simulink model "FOC"  (R2023a)
settings: Solver=ode1  StartTime=0.0  StopTime=0.2  FixedStep=ctrlConst.TsSwitch  MaxStep=1e-6  RelTol=1e-3  EnableMultiTasking=on
values from neighbouring files (symbols this model uses):
  f32_P_AngleCompCur = 5461.0    [bldc.sldd]
  f32_P_AngleCompVol = 1.5    [bldc.sldd]
  f32_P_IdInIF_A = -5.0    [bldc.sldd]
  f32_P_Modulation = 0.95    [bldc.sldd]
  u16_P_MotorPair = 4.0    [bldc.sldd]
undefined symbols (not defined in the file or in its folder): ECM, f32_P_Coef, FFW_enable, g_msgCore0to2_AcrKi, g_msgCore0to2_AcrKiStb, g_msgCore0to2_AcrKp, g_msgCore0to2_AcrKpStb, g_msgCore0to2_AcrSwtHiRpm, g_msgCore0to2_AcrSwtLoRpm, g_msgCore0to2_AfrKp, g_msgCore0to2_AfrTi, g_msgCore0to2_arc_dd_fi, g_msgCore0to2_CalibEn, g_msgCore0to2_clpwitch, g_msgCore0to2_DecoupleEn, g_msgCore0to2_dqLpf, g_msgCore0to2_dqLpfSpdCoef, g_msgCore0to2_FFW_Gain, g_msgCore0to2_linearKpEn, g_msgCore0to2_maxCur, g_msgCore0to2_maxFwcCurRatio, g_msgCore0to2_motorseq, g_msgCore0to2_MTPA_Gain, g_msgCore0to2_pwmFrqSet, g_msgCore0to2_spdswitch, IdROL_C, PWMFrqSwitch_C, SC_Ld_P, SC_Lq_P, SC_Psi_P, Tsw
libraries: MathLib x6, simulink x1
(part 2 of 2)

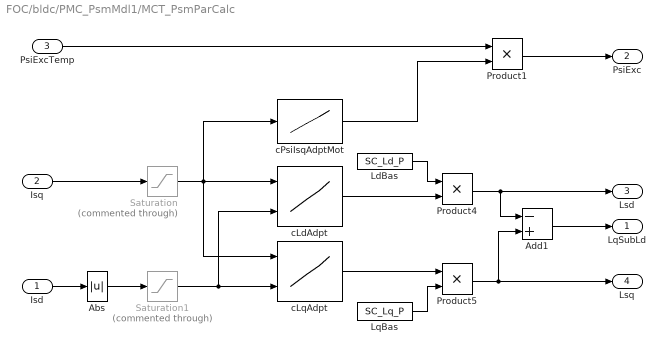
== system FOC/bldc/PMC_PsmMdl1/MCT_PsmParCalc ==
  Isd : Inport
  Isq : Inport  Port=2
  PsiExcTemp : Inport  Port=3
  Abs : Abs  SaturateOnIntegerOverflow=off
  Add1 : Sum  Inputs=-+
  LdBas : Constant  Value=SC_Ld_P  OutDataTypeStr=single  SampleTime=-1
  LqBas : Constant  Value=SC_Lq_P  OutDataTypeStr=single  SampleTime=-1
  Product1 : Product  OutDataTypeStr=single  RndMeth=Zero
  Product4 : Product  RndMeth=Zero  OutDataTypeStr=Inherit: Same as first input
  Product5 : Product  OutDataTypeStr=single  RndMeth=Zero
  Saturation : Saturate  Commented=through  UpperLimit=450  LowerLimit=-450
  Saturation1 : Saturate  Commented=through  UpperLimit=450  LowerLimit=0
  cLdAdpt : Lookup_n-D  DataSpecification=Lookup table object  LookupTableObject=cLdAdptMon_T  BreakpointsForDimension1=|  BreakpointsForDimension2=|  BeginIndexSearchUsingPreviousIndexResult=on  Table=|  ExtrapMethod=Clip  UseLastTableValue=on  InternalRulePriority=Speed  OutDataTypeStr=Inherit: Inherit from 'Table data'  InputSameDT=off
      BreakpointsForDimension1=|
      | [-530.4101839
      | -495.049505
      | -459.688826
      | -424.3281471
      | -388.9674682
      | -353.6067893
      | -318.2461103
      | -282.8854314
      | -247.5247525
      | -212.1640736
      | -176.8033946
      | -141.4427157
      | -106.0820368
      | -70.72135785
      | -35.36067893
      | 0
      | 35.36067893
      | 70.72135785
      | 106.0820368
      | 141.4427157
      | 176.8033946
      | 212.1640736
      | 247.5247525
      | 282.8854314
      | 318.2461103
      | 353.6067893
      | 388.9674682
      | 424.3281471
      | 459.688826
      | 495.049505
      | 530.4101839
      | ]
      BreakpointsForDimension2=|
      | [0	35.36067893	70.72135785	106.0820368	141.4427157	176.8033946	212.1640736	247.5247525	282.8854314	318.2461103	353.6067893	388.9674682	424.3281471	459.688826	495.049505	530.4101839
      | ]
      Table=|
      | [1	1	0.797297297	0.72972973	0.692567568	0.667567568	0.653153153	0.640926641	0.631756757	0.624624625	0.618918919	0.614742015	0.611486486	0.608731809	0.606177606	0.606177606
      | 1	1	0.797297297	0.72972973	0.692567568	0.667567568	0.653153153	0.640926641	0.631756757	0.624624625	0.618918919	0.614742015	0.611486486	0.608731809	0.606177606	0.606177606
      | 0.905405405	0.905405405	0.756756757	0.702702703	0.675675676	0.659459459	0.648648649	0.638996139	0.631756757	0.626126126	0.622972973	0.62002457	0.61768018	0.615800416	0.613899614	0.613899614
      | 0.810810811	0.810810811	0.716216216	0.68018018	0.665540541	0.651351351	0.644144144	0.638996139	0.633445946	0.630630631	0.628378378	0.626658477	0.625337838	0.624220374	0.622586873	0.622586873
      | 0.72972973	0.72972973	0.682432432	0.666666667	0.655405405	0.651351351	0.646396396	0.640926641	0.640202703	0.638138138	0.637027027	0.636240786	0.635585586	0.634927235	0.634169884	0.634169884
      | 0.635135135	0.635135135	0.648648649	0.648648649	0.648648649	0.648648649	0.646396396	0.646718147	0.64527027	0.645645646	0.646216216	0.646314496	0.646283784	0.646153846	0.645752896	0.645752896
      | 0.567567568	0.567567568	0.621621622	0.63963964	0.64527027	0.648648649	0.650900901	0.652509653	0.655405405	0.656606607	0.657837838	0.658562654	0.659009009	0.659043659	0.659266409	0.659266409
      | 0.513513514	0.513513514	0.601351351	0.630630631	0.64527027	0.654054054	0.65990991	0.664092664	0.665540541	0.67042042	0.672297297	0.673464373	0.674099099	0.674636175	0.673745174	0.673745174
      | 0.459459459	0.459459459	0.587837838	0.630630631	0.652027027	0.664864865	0.673423423	0.67953668	0.684121622	0.686786787	0.688918919	0.69017199	0.690653153	0.69022869	0.689189189	0.689189189
      | 0.432432432	0.432432432	0.587837838	0.63963964	0.668918919	0.683783784	0.695945946	0.702702703	0.706081081	0.709159159	0.710513514	0.713022113	0.710247748	0.708939709	0.707528958	0.707528958
      | 0.432432432	0.432432432	0.608108108	0.666666667	0.695945946	0.713513514	0.725225225	0.72972973	0.733108108	0.733483483	0.732986486	0.731572482	0.72972973	0.726611227	0.722972973	0.722972973
      | 0.486486486	0.486486486	0.662162162	0.716216216	0.743243243	0.754054054	0.761261261	0.760617761	0.760304054	0.758108108	0.755135135	0.751474201	0.747747748	0.742203742	0.737451737	0.737451737
      | 0.594594595	0.594594595	0.736486486	0.774774775	0.787162162	0.789189189	0.788288288	0.785714286	0.781756757	0.777027027	0.771891892	0.766093366	0.760135135	0.753638254	0.747104247	0.747104247
      | 0.72972973	0.72972973	0.804054054	0.81981982	0.820945946	0.818918919	0.813063063	0.806949807	0.8	0.792747748	0.78527027	0.777641278	0.77027027	0.761954262	0.754826255	0.754826255
      | 0.797297297	0.797297297	0.837837838	0.842342342	0.841216216	0.835135135	0.826576577	0.82046332	0.81097973	0.802012012	0.792837838	0.783783784	0.774774775	0.767151767	0.758687259	0.758687259
      | 0.790540541	0.790540541	0.834459459	0.84009009	0.837837838	0.832432432	0.82545045	0.818532819	0.809712838	0.800848348	0.791756757	0.782555283	0.774211712	0.766112266	0.757722008	0.757722008
      | 0.783783784	0.783783784	0.831081081	0.837837838	0.834459459	0.82972973	0.824324324	0.816602317	0.808445946	0.799684685	0.790675676	0.781326781	0.773648649	0.765072765	0.756756757	0.756756757
      | 0.689189189	0.689189189	0.783783784	0.806306306	0.810810811	0.810810811	0.806306306	0.801158301	0.794932432	0.788243243	0.781216216	0.773710074	0.765765766	0.758835759	0.751930502	0.751930502
      | 0.554054054	0.554054054	0.716216216	0.756756757	0.773648649	0.781081081	0.781531532	0.77992278	0.776013514	0.771921922	0.767162162	0.761793612	0.755630631	0.749480249	0.744208494	0.744208494
      | 0.418918919	0.418918919	0.628378378	0.693693694	0.726351351	0.743243243	0.75	0.752895753	0.752195946	0.750900901	0.748513514	0.745331695	0.742117117	0.737006237	0.732625483	0.732625483
      | 0.351351351	0.351351351	0.567567568	0.63963964	0.675675676	0.697297297	0.709459459	0.718146718	0.722972973	0.724024024	0.736459459	0.723587224	0.721846847	0.719334719	0.716216216	0.716216216
      | 0.351351351	0.351351351	0.547297297	0.612612613	0.64527027	0.664864865	0.677927928	0.687258687	0.694256757	0.697747748	0.7	0.701105651	0.701238739	0.700623701	0.698841699	0.698841699
      | 0.378378378	0.378378378	0.547297297	0.599099099	0.628378378	0.662162162	0.657657658	0.666023166	0.670608108	0.675375375	0.678378378	0.68034398	0.681418919	0.681912682	0.681467181	0.681467181
      | 0.405405405	0.405405405	0.547297297	0.594594595	0.618243243	0.632432432	0.641891892	0.646718147	0.652027027	0.656306306	0.659189189	0.661277641	0.662725225	0.663201663	0.664092664	0.664092664
      | 0.459459459	0.459459459	0.560810811	0.599099099	0.614864865	0.624324324	0.630630631	0.635135135	0.638513514	0.641141141	0.643648649	0.64546683	0.646734234	0.647609148	0.647683398	0.647683398
      | 0.513513514	0.513513514	0.587837838	0.608108108	0.614864865	0.618918919	0.623873874	0.625482625	0.628378378	0.629129129	0.631216216	0.632309582	0.633220721	0.633783784	0.634169884	0.634169884
      | 0.594594595	0.594594595	0.614864865	0.621621622	0.621621622	0.621621622	0.619369369	0.61969112	0.619932432	0.62012012	0.621081081	0.621498771	0.621734234	0.621933472	0.621621622	0.621621622
      | 0.675675676	0.675675676	0.641891892	0.635135135	0.628378378	0.624324324	0.619369369	0.617760618	0.614864865	0.614114114	0.612837838	0.612285012	0.611936937	0.611538462	0.611003861	0.611003861
      | 0.756756757	0.756756757	0.682432432	0.653153153	0.638513514	0.62972973	0.621621622	0.615830116	0.611486486	0.608108108	0.606351351	0.604545455	0.603502252	0.602494802	0.601640927	0.601640927
      | 0.851351351	0.851351351	0.716216216	0.675675676	0.652027027	0.635135135	0.623873874	0.615830116	0.609797297	0.605105105	0.601216216	0.598525799	0.596418919	0.594698545	0.593243243	0.593243243
      | 0.851351351	0.851351351	0.716216216	0.675675676	0.652027027	0.635135135	0.623873874	0.615830116	0.609797297	0.605105105	0.601216216	0.598525799	0.596418919	0.594698545	0.593243243	0.593243243
      | ]
      settings: InputPortMap=u0,u1
  cLqAdpt : Lookup_n-D  DataSpecification=Lookup table object  LookupTableObject=cLqAdptMon_T  BreakpointsForDimension1=|  BreakpointsForDimension2=|  BeginIndexSearchUsingPreviousIndexResult=on  Table=|  ExtrapMethod=Clip  UseLastTableValue=on  InternalRulePriority=Speed  OutDataTypeStr=Inherit: Inherit from 'Table data'  InputSameDT=off
      BreakpointsForDimension1=|
      | [-530.4101839
      | -495.049505
      | -459.688826
      | -424.3281471
      | -388.9674682
      | -353.6067893
      | -318.2461103
      | -282.8854314
      | -247.5247525
      | -212.1640736
      | -176.8033946
      | -141.4427157
      | -106.0820368
      | -70.72135785
      | -35.36067893
      | 0
      | 35.36067893
      | 70.72135785
      | 106.0820368
      | 141.4427157
      | 176.8033946
      | 212.1640736
      | 247.5247525
      | 282.8854314
      | 318.2461103
      | 353.6067893
      | 388.9674682
      | 424.3281471
      | 459.688826
      | 495.049505
      | 530.4101839
      | ]
      BreakpointsForDimension2=|
      | [0	35.36067893	70.72135785	106.0820368	141.4427157	176.8033946	212.1640736	247.5247525	282.8854314	318.2461103	353.6067893	388.9674682	424.3281471	459.688826	495.049505	530.4101839
      | ]
      Table=|
      | [0.394500897	0.39748954	0.39748954	0.400478183	0.403466826	0.403466826	0.403466826	0.406455469	0.406455469	0.406455469	0.403466826	0.403466826	0.403466826	0.400478183	0.400478183	0.400478183
      | 0.394500897	0.39748954	0.39748954	0.400478183	0.403466826	0.403466826	0.403466826	0.406455469	0.406455469	0.406455469	0.403466826	0.403466826	0.403466826	0.400478183	0.400478183	0.400478183
      | 0.418410042	0.421628581	0.424847119	0.424847119	0.428065658	0.428065658	0.428065658	0.428065658	0.431284197	0.428065658	0.428065658	0.428065658	0.424847119	0.424847119	0.421628581	0.421628581
      | 0.446304045	0.449790795	0.453277545	0.453277545	0.456764296	0.456764296	0.456764296	0.456764296	0.456764296	0.456764296	0.453277545	0.453277545	0.449790795	0.449790795	0.446304045	0.446304045
      | 0.479269684	0.483073412	0.483073412	0.48687714	0.48687714	0.48687714	0.48687714	0.48687714	0.48687714	0.48687714	0.483073412	0.483073412	0.479269684	0.475465957	0.471662229	0.471662229
      | 0.514644351	0.518828452	0.518828452	0.523012552	0.523012552	0.523012552	0.523012552	0.523012552	0.523012552	0.518828452	0.514644351	0.514644351	0.510460251	0.506276151	0.49790795	0.49790795
      | 0.557880056	0.562529056	0.562529056	0.562529056	0.562529056	0.562529056	0.562529056	0.562529056	0.557880056	0.557880056	0.553231055	0.548582055	0.543933054	0.534635053	0.529986053	0.529986053
      | 0.606694561	0.611924686	0.611924686	0.611924686	0.611924686	0.611924686	0.606694561	0.606694561	0.601464435	0.59623431	0.591004184	0.585774059	0.575313808	0.570083682	0.559623431	0.559623431
      | 0.669456067	0.669456067	0.669456067	0.669456067	0.669456067	0.663478781	0.663478781	0.657501494	0.651524208	0.639569635	0.633592349	0.621637776	0.61566049	0.603705918	0.593544531	0.593544531
      | 0.739191074	0.739191074	0.739191074	0.732217573	0.732217573	0.725244073	0.718270572	0.711297071	0.69735007	0.686889819	0.675034868	0.663179916	0.650627615	0.637377964	0.624825662	0.624825662
      | 0.816736402	0.815899582	0.812552301	0.806694561	0.79748954	0.785774059	0.772384937	0.758158996	0.743933054	0.728870293	0.713807531	0.69790795	0.682845188	0.667782427	0.652719665	0.652719665
      | 0.900627615	0.894351464	0.882845188	0.868200837	0.851464435	0.833682008	0.815899582	0.79707113	0.779288703	0.761506276	0.743723849	0.725941423	0.708158996	0.691422594	0.675732218	0.675732218
      | 0.965132497	0.949790795	0.928870293	0.907949791	0.885634589	0.864714086	0.845188285	0.824267782	0.80334728	0.782426778	0.762900976	0.741980474	0.723849372	0.705718271	0.688981869	0.688981869
      | 0.991631799	0.972803347	0.951882845	0.930962343	0.907949791	0.887029289	0.864016736	0.838912134	0.815899582	0.728033473	0.769874477	0.748953975	0.728033473	0.709205021	0.690376569	0.690376569
      | 1	0.979079498	0.958158996	0.937238494	0.920502092	0.89539749	0.866108787	0.841004184	0.811715481	0.786610879	0.757322176	0.736401674	0.715481172	0.690376569	0.673640167	0.673640167
      | 1	0.981171548	0.964435146	0.947698745	0.933054393	0.910041841	0.884937238	0.861924686	0.836820084	0.813807531	0.790794979	0.771966527	0.755230126	0.734309623	0.719665272	0.719665272
      | 1	0.983263598	0.970711297	0.958158996	0.945606695	0.924686192	0.90376569	0.882845188	0.861924686	0.841004184	0.824267782	0.807531381	0.794979079	0.778242678	0.765690377	0.765690377
      | 0.991631799	0.951882845	0.958158996	0.939330544	0.920502092	0.90167364	0.882845188	0.861924686	0.841004184	0.820083682	0.80125523	0.784518828	0.767782427	0.751046025	0.738493724	0.738493724
      | 0.965132497	0.951185495	0.933054393	0.913528591	0.894002789	0.875871688	0.857740586	0.839609484	0.820083682	0.80195258	0.783821478	0.767085077	0.750348675	0.735006974	0.719665272	0.719665272
      | 0.900627615	0.896443515	0.887029289	0.873430962	0.857740586	0.842050209	0.825313808	0.808577406	0.791841004	0.776150628	0.759414226	0.743723849	0.728033473	0.712343096	0.697698745	0.697698745
      | 0.816736402	0.817573222	0.815062762	0.810041841	0.80167364	0.791631799	0.779916318	0.767364017	0.753974895	0.739748954	0.725523013	0.711297071	0.69790795	0.683682008	0.670292887	0.670292887
      | 0.739191074	0.739191074	0.739191074	0.739191074	0.732217573	0.732217573	0.725244073	0.711297071	0.70432357	0.69525802	0.684797768	0.673640167	0.661785216	0.649930265	0.638075314	0.638075314
      | 0.669456067	0.669456067	0.669456067	0.669456067	0.669456067	0.669456067	0.663478781	0.657501494	0.657501494	0.645546922	0.639569635	0.633592349	0.621637776	0.61566049	0.603705918	0.603705918
      | 0.606694561	0.611924686	0.611924686	0.611924686	0.611924686	0.611924686	0.611924686	0.611924686	0.606694561	0.601464435	0.59623431	0.591004184	0.585774059	0.575313808	0.570083682	0.570083682
      | 0.557880056	0.562529056	0.562529056	0.567178057	0.567178057	0.567178057	0.567178057	0.562529056	0.562529056	0.557880056	0.557880056	0.553231055	0.548582055	0.543933054	0.539284054	0.539284054
      | 0.514644351	0.518828452	0.518828452	0.523012552	0.523012552	0.527196653	0.527196653	0.527196653	0.523012552	0.523012552	0.518828452	0.518828452	0.514644351	0.510460251	0.506276151	0.506276151
      | 0.479269684	0.479269684	0.483073412	0.48687714	0.48687714	0.490680867	0.490680867	0.490680867	0.490680867	0.490680867	0.48687714	0.48687714	0.483073412	0.479269684	0.475465957	0.475465957
      | 0.446304045	0.449790795	0.453277545	0.453277545	0.456764296	0.456764296	0.456764296	0.460251046	0.460251046	0.460251046	0.456764296	0.456764296	0.453277545	0.453277545	0.449790795	0.449790795
      | 0.418410042	0.421628581	0.424847119	0.424847119	0.428065658	0.428065658	0.431284197	0.431284197	0.431284197	0.431284197	0.431284197	0.431284197	0.428065658	0.428065658	0.424847119	0.424847119
      | 0.394500897	0.39748954	0.39748954	0.400478183	0.403466826	0.403466826	0.406455469	0.406455469	0.406455469	0.406455469	0.406455469	0.406455469	0.406455469	0.403466826	0.403466826	0.403466826
      | 0.394500897	0.39748954	0.39748954	0.400478183	0.403466826	0.403466826	0.406455469	0.406455469	0.406455469	0.406455469	0.406455469	0.406455469	0.406455469	0.403466826	0.403466826	0.403466826
      | ]
      settings: InputPortMap=u0,u1
  cPsiIsqAdptMot : Lookup_n-D  NumberOfTableDimensions=1  DataSpecification=Lookup table object  LookupTableObject=cPsiIsqAdptMot_TT  BreakpointsForDimension1=|  BeginIndexSearchUsingPreviousIndexResult=on  Table=|  ExtrapMethod=Clip  UseLastTableValue=on  InternalRulePriority=Speed  OutDataTypeStr=Inherit: Inherit from 'Table data'
      BreakpointsForDimension1=|
      | [-530.4101839
      | -495.049505
      | -459.688826
      | -424.3281471
      | -388.9674682
      | -353.6067893
      | -318.2461103
      | -282.8854314
      | -247.5247525
      | -212.1640736
      | -176.8033946
      | -141.4427157
      | -106.0820368
      | -70.72135785
      | -35.36067893
      | 0
      | 35.36067893
      | 70.72135785
      | 106.0820368
      | 141.4427157
      | 176.8033946
      | 212.1640736
      | 247.5247525
      | 282.8854314
      | 318.2461103
      | 353.6067893
      | 388.9674682
      | 424.3281471
      | 459.688826
      | 495.049505
      | 530.4101839
      | ]
      Table=|
      | [0.983333333
      | 0.983333333
      | 0.985185185
      | 0.987037037
      | 0.990740741
      | 0.992592593
      | 0.994444444
      | 0.996296296
      | 0.996296296
      | 0.998148148
      | 0.998148148
      | 0.998148148
      | 0.994444444
      | 0.992592593
      | 0.990740741
      | 0.990740741
      | 0.990740741
      | 0.992592593
      | 0.996296296
      | 1
      | 1
      | 1
      | 1
      | 0.998148148
      | 0.996296296
      | 0.994444444
      | 0.992592593
      | 0.990740741
      | 0.988888889
      | 0.987037037
      | 0.987037037]
  LqSubLd : Outport  VectorParamsAs1DForOutWhenUnconnected=off
  PsiExc : Outport  Port=2  VectorParamsAs1DForOutWhenUnconnected=off
  Lsd : Outport  Port=3  VectorParamsAs1DForOutWhenUnconnected=off
  Lsq : Outport  Port=4  VectorParamsAs1DForOutWhenUnconnected=off
  wires:
  PsiExcTemp/1 -> Product1/1
  Add1/1 -> LqSubLd/1
  Product5/1 -> Add1/2, Lsq/1
  Product4/1 -> Add1/1, Lsd/1
  Product1/1 -> PsiExc/1
  LqBas/1 -> Product5/2
  cLqAdpt/1 -> Product5/1
  cLdAdpt/1 -> Product4/2
  LdBas/1 -> Product4/1
  Abs/1 -> Saturation1/1
  Isq/1 -> Saturation/1
  Isd/1 -> Abs/1
  cPsiIsqAdptMot/1 -> Product1/2
  Saturation/1 -> cLqAdpt/1, cLdAdpt/1, cPsiIsqAdptMot/1
  Saturation1/1 -> cLqAdpt/2, cLdAdpt/2

== system FOC/bldc/PMC_PsmMdl1/PMC_TrqCal ==
  PMC_LqSubLd : Inport
  PMC_PsiExc : Inport  Port=2
  MCT_isdFlt : Inport  Port=3
  MCT_isqFlt : Inport  Port=4
  Constant : Constant  Value=500  OutDataTypeStr=single
  Gain1 : Gain  Gain=3*u16_P_MotorPair
  Gain2 : Gain  Gain=-1  ParamDataTypeStr=single
  Product : Product
  Product1 : Product
  Product2 : Product
  Saturation Dynamic1 : simulink/Discontinuities/Saturation Dynamic  OutMin=[]  OutMax=[]  OutDataTypeStr=Inherit: Same as second input  OutDataType=fixdt(1, 16)  OutScaling=2^-10  DoSatur=off
  Sum : Sum  Inputs=|+-
  MCT_TrqAct : Outport  VectorParamsAs1DForOutWhenUnconnected=off
  wires:
  Saturation Dynamic1/1 -> MCT_TrqAct/1
  Gain1/1 -> Saturation Dynamic1/2
  Constant/1 -> Saturation Dynamic1/1, Gain2/1
  Gain2/1 -> Saturation Dynamic1/3
  Sum/1 -> Gain1/1
  MCT_isqFlt/1 -> Product/2, Product2/1
  PMC_PsiExc/1 -> Product/1
  Product/1 -> Sum/1
  PMC_LqSubLd/1 -> Product1/2
  MCT_isdFlt/1 -> Product1/1
  Product1/1 -> Product2/2
  Product2/1 -> Sum/2

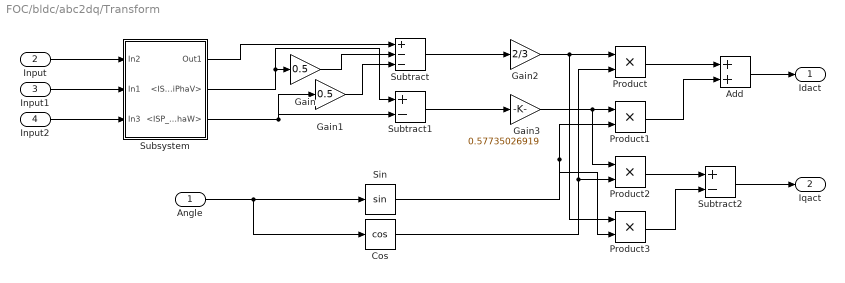
== system FOC/bldc/abc2dq/Transform ==
  Angle : Inport
  Input : Inport  Port=2
  Input1 : Inport  Port=3
  Input2 : Inport  Port=4
  Add : Sum  OutDataTypeStr=single
  Cos : Trigonometry  Operator=cos  OutputSignalType=real
  Gain : Gain  Gain=0.5
  Gain1 : Gain  Gain=0.5
  Gain2 : Gain  Gain=2/3
  Gain3 : Gain  Gain=0.57735026919
  Product{,1..3} (4 alike) : Product
  Sin : Trigonometry
  Subsystem : Subsystem
  Subtract : Sum  Inputs=+--
  Subtract1 : Sum  Inputs=+-
  Subtract2 : Sum  Inputs=+-  OutDataTypeStr=single
  Idact : Outport
  Iqact : Outport  Port=2
  wires:
  Subsystem/1(Out1) -> Subtract/1
  Subsystem/2(<ISP_iPhaV>) -> Subtract1/1, Gain/1
  Subsystem/3(<ISP_iPhaW>) -> Gain1/1, Subtract1/2
  Gain/1 -> Subtract/2
  Gain1/1 -> Subtract/3
  Subtract/1 -> Gain2/1
  Subtract1/1 -> Gain3/1
  Gain2/1 -> Product3/1, Product/1
  Cos/1 -> Product2/2, Product/2
  Product/1 -> Add/1
  Gain3/1 -> Product2/1, Product1/1
  Product1/1 -> Add/2
  Add/1 -> Idact/1
  Product2/1 -> Subtract2/1
  Product3/1 -> Subtract2/2
  Subtract2/1 -> Iqact/1
  Angle/1 -> Sin/1, Cos/1
  Sin/1 -> Product3/2, Product1/2
  Input1/1 -> Subsystem/2(In1)
  Input/1 -> Subsystem/1(In2)
  Input2/1 -> Subsystem/3(In3)

== system FOC/bldc/PMC_IsDesCalc/FWC/PI ==
  error : Inport
  Ts : Inport  Port=2
  Constant : Constant  Value=0.25  OutDataTypeStr=single
  Constant1 : Constant  Value=g_msgCore0to2_AfrKp
  Constant2 : Constant  Value=1.0  OutDataTypeStr=single
  Constant4 : Constant  Value=g_msgCore0to2_maxCur  OutDataTypeStr=single
  Constant5 : Constant  Value=g_msgCore0to2_AfrTi
  Constant6 : Constant  Value=0  OutDataTypeStr=single
  Divide : Product  Inputs=**  OutDataTypeStr=single
  Divide1 : Product  Inputs=**/  OutDataTypeStr=single
  Divide2 : Product  Inputs=**  OutDataTypeStr=single
  Divide3 : Product  Inputs=**  OutDataTypeStr=single
  Switch : Switch  Criteria=u2 > Threshold  SaturateOnIntegerOverflow=off  InputSameDT=off
  Switch2 : Switch  Criteria=u2 ~= 0  SaturateOnIntegerOverflow=off  InputSameDT=off
  Kp : Outport  VectorParamsAs1DForOutWhenUnconnected=off
  Ki : Outport  Port=2  VectorParamsAs1DForOutWhenUnconnected=off
  wires:
  Constant/1 -> Switch/1
  error/1 -> Switch/2
  Constant1/1 -> Divide/1
  Constant4/1 -> Divide/2
  Divide/1 -> Divide2/1, Divide1/1
  Ts/1 -> Divide1/2
  Constant5/1 -> Switch2/2, Divide1/3
  Divide1/1 -> Switch2/1
  Constant6/1 -> Switch2/3
  Switch2/1 -> Divide3/1
  Constant2/1 -> Switch/3
  Switch/1 -> Divide3/2, Divide2/2
  Divide2/1 -> Kp/1
  Divide3/1 -> Ki/1

== system FOC/bldc/PMC_IsDesCalc/MaxI vs Freq/PT1_2 ==
  bin : Inport
  cof : Inport  Port=2
  Constant : Constant  OutDataTypeStr=single
  Product1 : Product  RndMeth=Zero  OutDataTypeStr=Inherit: Same as first input
  Product3 : Product  RndMeth=Zero  OutDataTypeStr=Inherit: Same as first input
  Subtract : Sum  Inputs=-+  OutDataTypeStr=Inherit: Same as first input
  Sum1 : Sum  Inputs=|++  OutDataTypeStr=Inherit: Same as first input
  Unit Delay1 : UnitDelay  SampleTime=-1  HasFrameUpgradeWarning=on
  bout : Outport  VectorParamsAs1DForOutWhenUnconnected=off
  wires:
  Subtract/1 -> Product3/2
  Sum1/1 -> Unit Delay1/1, bout/1
  cof/1 -> Product1/2, Subtract/1
  Constant/1 -> Subtract/2
  bin/1 -> Product1/1
  Product1/1 -> Sum1/1
  Unit Delay1/1 -> Product3/1
  Product3/1 -> Sum1/2

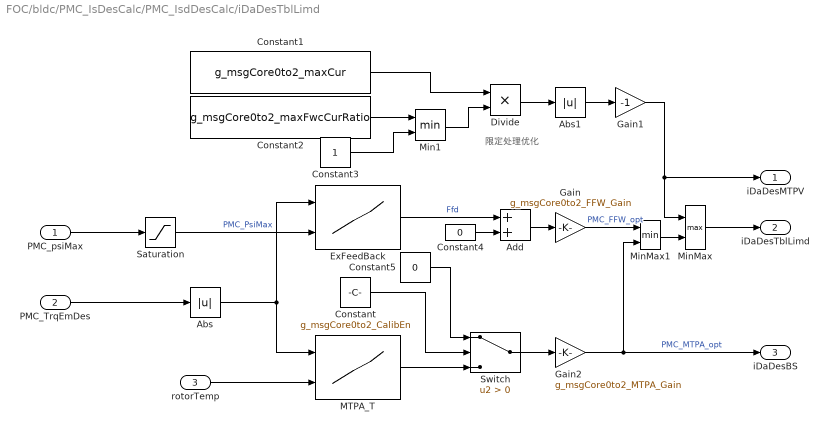
== system FOC/bldc/PMC_IsDesCalc/PMC_IsdDesCalc/iDaDesTblLimd ==
  note: 限定处理优化
  PMC_psiMax : Inport
  PMC_TrqEmDes : Inport  Port=2
  rotorTemp : Inport  Port=3
  Abs : Abs  SaturateOnIntegerOverflow=off
  Abs1 : Abs  OutDataTypeStr=single  SaturateOnIntegerOverflow=off
  Add : Sum
  Constant : Constant  Value=g_msgCore0to2_CalibEn
  Constant1 : Constant  Value=g_msgCore0to2_maxCur  OutDataTypeStr=single
  Constant2 : Constant  Value=g_msgCore0to2_maxFwcCurRatio  OutDataTypeStr=single
  Constant3 : Constant  OutDataTypeStr=single
  Constant4 : Constant  Value=0  OutDataTypeStr=single  SampleTime=-1
  Constant5 : Constant  Value=0  OutDataTypeStr=single
  Divide : Product  Inputs=**  OutDataTypeStr=single
  ExFeedBack : Lookup_n-D  DataSpecification=Lookup table object  LookupTableObject=ExFeedBack_T  BreakpointsForDimension1=|  BreakpointsForDimension2=|  BeginIndexSearchUsingPreviousIndexResult=on  Table=|  ExtrapMethod=Clip  UseLastTableValue=on  InternalRulePriority=Speed  OutDataTypeStr=Inherit: Inherit from 'Table data'  RndMeth=Simplest
      BreakpointsForDimension1=|
      | [0.015
      | 0.02
      | 0.025
      | 0.03
      | 0.035
      | 0.04
      | 0.06
      | 0.09]
      Table=|
      | [-180	-205	-250	-325	-340	-340	-340	-340	-340	-340	-340	-340	-340	-340	-340	-340	-340	-340	-340	-340	-340
      | -140	-160	-200	-255	-325	-340	-340	-340	-340	-340	-340	-340	-340	-340	-340	-340	-340	-340	-340	-340	-340
      | -100	-120	-160	-205	-275	-325	-340	-340	-340	-340	-340	-340	-340	-340	-340	-340	-340	-340	-340	-340	-340
      | -55	-80	-125	-170	-215	-280	-325	-340	-340	-340	-340	-340	-340	-340	-340	-340	-340	-340	-340	-340	-340
      | -20	-50	-90	-135	-180	-230	-295	-340	-340	-340	-340	-340	-340	-340	-340	-340	-340	-340	-340	-340	-340
      | -10	-20	-65	-105	-150	-190	-230	-280	-325	-340	-340	-340	-340	-340	-340	-340	-340	-340	-340	-340	-340
      | 0	-10	-30	-47	-60	-80	-115	-150	-180	-215	-245	-290	-325	-340	-340	-340	-340	-340	-340	-340	-340
      | 0	-10	-30	-47	-60	-78	-98	-113	-132	-152	-172	-194	-214	-228	-247	-271	-291	-315	-340	-340	-340
      | ]
      BreakpointsForDimension2=|
      | [0	20	40	60	80	100	120	140	160	180	200	220	240	260	280	300	320	340	360	380	400
      | ]
      settings: InputPortMap=u0,u1
  Gain : Gain  Gain=g_msgCore0to2_FFW_Gain
  Gain1 : Gain  Gain=-1  OutDataTypeStr=single
  Gain2 : Gain  Gain=g_msgCore0to2_MTPA_Gain
  MTPA_T : Lookup_n-D  DataSpecification=Lookup table object  LookupTableObject=MTPA_T  BreakpointsForDimension1=|  BreakpointsForDimension2=|  BeginIndexSearchUsingPreviousIndexResult=on  Table=|  ExtrapMethod=Clip  UseLastTableValue=on  InternalRulePriority=Speed  OutDataTypeStr=Inherit: Inherit from 'Table data'  RndMeth=Simplest
      BreakpointsForDimension1=|
      | [0
      | 20
      | 40
      | 60
      | 80
      | 100
      | 120
      | 140
      | 160
      | 180
      | 200
      | 220
      | 240
      | 260
      | 280
      | 300
      | 320
      | 340
      | 360
      | 380
      | 400]
      Table=|
      | [0.0 	0.0 	0.0 	0.0 	0.0 	0.0 	0.0 
      | -11.0 	-12.0 	-13.0 	-14.1 	-15.1 	-16.2 	-17.0 
      | -21.0 	-23.2 	-25.4 	-27.6 	-29.8 	-32.2 	-34.0 
      | -35.0 	-37.5 	-40.1 	-44.0 	-45.2 	-48.0 	-50.0 
      | -50.0 	-52.9 	-55.8 	-58.6 	-61.5 	-64.7 	-67.0 
      | -61.0 	-65.2 	-69.5 	-72.0 	-77.9 	-82.6 	-86.0 
      | -75.0 	-79.9 	-84.8 	-89.7 	-94.7 	-100.1 	-104.0 
      | -89.0 	-95.1 	-101.2 	-107.0 	-113.4 	-120.1 	-125.0 
      | -104.0 	-111.1 	-118.2 	-125.4 	-132.5 	-140.3 	-146.0 
      | -123.0 	-129.9 	-136.9 	-145.0 	-150.8 	-158.4 	-164.0 
      | -141.0 	-150.0 	-157.0 	-164.0 	-170.1 	-179.0 	-184.0 
      | -160.0 	-168.0 	-175.9 	-185.0 	-191.9 	-200.6 	-207.0 
      | -179.0 	-187.5 	-195.9 	-204.4 	-212.9 	-222.2 	-229.0 
      | -193.0 	-202.7 	-212.3 	-222.0 	-231.6 	-242.3 	-250.0 
      | -212.0 	-222.0 	-232.0 	-242.0 	-252.0 	-263.0 	-271.0 
      | -230.0 	-241.0 	-252.0 	-257.0 	-274.1 	-286.2 	-295.0 
      | -248.0 	-259.7 	-271.4 	-279.0 	-294.8 	-307.7 	-317.0 
      | -269.0 	-280.0 	-289.0 	-301.0 	-317.0 	-334.0 	-342.0 
      | -288.0 	-300.5 	-313.1 	-327.0 	-342.0 	-352.0 	-362.0 
      | -303.0 	-316.7 	-330.5 	-348.0 	-357.9 	-373.0 	-384.0 
      | -320.0 	-335.3 	-350.5 	-372.0 	-381.0 	-397.8 	-410.0 ]
      BreakpointsForDimension2=|
      | [-40	0	40	80	120	160	180
      | ]
      settings: InputPortMap=u0,u1
  Min1 : MinMax  Inputs=2
  MinMax : MinMax  Function=max  Inputs=2
  MinMax1 : MinMax  Inputs=2
  Saturation : Saturate  UpperLimit=0.18  LowerLimit=0.006
  Switch : Switch  Criteria=u2 > Threshold  SaturateOnIntegerOverflow=off  InputSameDT=off
  iDaDesMTPV : Outport  VectorParamsAs1DForOutWhenUnconnected=off
  iDaDesTblLimd : Outport  Port=2  VectorParamsAs1DForOutWhenUnconnected=off
  iDaDesBS : Outport  Port=3  VectorParamsAs1DForOutWhenUnconnected=off
  wires:
  Gain1/1 -> MinMax/1, iDaDesMTPV/1
  Constant4/1 -> Add/2
  ExFeedBack/1 -> Add/1  "Ffd"
  Switch/1 -> Gain2/1
  PMC_TrqEmDes/1 -> Abs/1
  MinMax/1 -> iDaDesTblLimd/1
  MinMax1/1 -> MinMax/2
  Saturation/1 -> ExFeedBack/2  "PMC_PsiMax"
  PMC_psiMax/1 -> Saturation/1
  Abs/1 -> ExFeedBack/1, MTPA_T/1
  rotorTemp/1 -> MTPA_T/2
  Divide/1 -> Abs1/1
  Constant1/1 -> Divide/1
  Abs1/1 -> Gain1/1
  Constant3/1 -> Min1/2
  Min1/1 -> Divide/2
  Constant2/1 -> Min1/1
  Constant/1 -> Switch/2
  MTPA_T/1 -> Switch/3
  Constant5/1 -> Switch/1
  Add/1 -> Gain/1
  Gain/1 -> MinMax1/1  "PMC_FFW_opt"
  Gain2/1 -> MinMax1/2, iDaDesBS/1  "PMC_MTPA_opt"

== system FOC/bldc/PMC_IsDesCalc/PMC_IsqDesCalc/IsqDesLim_Calc ==
  IsqTrqDes : Inport
  MCT_IsdDes : Inport  Port=2
  MCT_sgnTrqEmDes : Inport  Port=3
  Ismax : Inport  Port=4
  IsResDes : Constant  Value=0  OutDataTypeStr=single  SampleTime=-1
  Math Function : Math  Operator=square  SignedPower=on
  Math Function1 : Math  Operator=square  SignedPower=on
  Math Function2 : Math  Operator=square  SignedPower=on
  Product : Product  Inputs=**  RndMeth=Zero
  Relational Operator : RelationalOperator  Operator=<=  OutDataTypeStr=boolean  InputSameDT=off
  SQRT : Subsystem
  Sum1 : Sum  Inputs=|+-
  Sum2 : Sum  Inputs=|+-
  bIsResLimActv : Outport  VectorParamsAs1DForOutWhenUnconnected=off
  IsqDesLim : Outport  Port=2  VectorParamsAs1DForOutWhenUnconnected=off
  wires:
  Product/1 -> IsqDesLim/1
  Relational Operator/1 -> SQRT/Enable, bIsResLimActv/1
  MCT_sgnTrqEmDes/1 -> Product/2
  SQRT/1(Sqrt1) -> Product/1
  Sum1/1 -> SQRT/1(x), Sum2/1
  IsResDes/1 -> Relational Operator/2
  Sum2/1 -> Relational Operator/1
  Math Function2/1 -> Sum2/2
  Math Function1/1 -> Sum1/2
  Math Function/1 -> Sum1/1
  IsqTrqDes/1 -> Math Function2/1
  MCT_IsdDes/1 -> Math Function1/1
  Ismax/1 -> Math Function/1

== system FOC/bldc/PMC_IsDesCalc/PMC_IsqDesCalc/IsqTrqDes_Calc ==
  MCT_TrqEmDes : Inport
  MCT_IsdDes : Inport  Port=2
  MCT_LqSubLd : Inport  Port=3
  MCT_PsiExc : Inport  Port=4
  Constant10 : Constant  Value=g_msgCore0to2_CalibEn
  MCT_PsmPsiTrqCalc : Subsystem
  MCT_TrqEmLos : Constant  Value=0  OutDataTypeStr=single
  Product : Product  Inputs=*/  RndMeth=Zero
  Sum3 : Sum  Inputs=|+-
  Switch : Switch  Criteria=u2 > Threshold  SaturateOnIntegerOverflow=off  InputSameDT=off
  IsqTrqDes : Outport  VectorParamsAs1DForOutWhenUnconnected=off
  LqsubLdId : Outport  Port=2
  psi : Outport  Port=3
  wires:
  MCT_IsdDes/1 -> MCT_PsmPsiTrqCalc/1(MCT_IsdDes)
  MCT_PsiExc/1 -> MCT_PsmPsiTrqCalc/3(MCT_PsiExc)
  MCT_LqSubLd/1 -> MCT_PsmPsiTrqCalc/2(MCT_LqSubLd)
  MCT_TrqEmLos/1 -> Sum3/2
  MCT_TrqEmDes/1 -> Sum3/1
  MCT_PsmPsiTrqCalc/1(psiMul3p) -> Product/2
  Constant10/1 -> Switch/2
  Switch/1 -> IsqTrqDes/1
  Product/1 -> Switch/3
  Sum3/1 -> Switch/1, Product/1
  MCT_PsmPsiTrqCalc/2(LqsubLdId) -> LqsubLdId/1
  MCT_PsmPsiTrqCalc/3(psi) -> psi/1

== system FOC/bldc/abc2dq/Transform/Subsystem ==
  In2 : Inport
  In1 : Inport  Port=2
  In3 : Inport  Port=3
  Constant : Constant  Value=g_msgCore0to2_motorseq  OutDataTypeStr=uint16
  Switch : Switch  Criteria=u2 > Threshold  SaturateOnIntegerOverflow=off  InputSameDT=off
  Switch1 : Switch  Criteria=u2 > Threshold  SaturateOnIntegerOverflow=off  InputSameDT=off
  Out1 : Outport
  <ISP_iPhaV> : Outport  Port=2
  <ISP_iPhaW> : Outport  Port=3
  wires:
  In2/1 -> Out1/1
  In1/1 -> Switch/3, Switch1/1
  Switch1/1 -> <ISP_iPhaV>/1
  In3/1 -> Switch1/3, Switch/1
  Constant/1 -> Switch/2, Switch1/2
  Switch/1 -> <ISP_iPhaW>/1

== system FOC/bldc/PMC_IsDesCalc/PMC_IsqDesCalc/IsqDesLim_Calc/SQRT ==
  x : Inport
  Enable : EnablePort
  Abs : Abs  SaturateOnIntegerOverflow=off
  Sqrt : Sqrt
  Sqrt1 : Outport  VectorParamsAs1DForOutWhenUnconnected=off
  wires:
  x/1 -> Abs/1
  Abs/1 -> Sqrt/1
  Sqrt/1 -> Sqrt1/1

== system FOC/bldc/PMC_IsDesCalc/PMC_IsqDesCalc/IsqTrqDes_Calc/MCT_PsmPsiTrqCalc ==
  MCT_IsdDes : Inport
  MCT_LqSubLd : Inport  Port=2
  MCT_PsiExc : Inport  Port=3
  3p : Constant  Value=u16_P_MotorPair*3  OutDataTypeStr=single
  Product1 : Product  Inputs=**  RndMeth=Zero
  Product2 : Product  Inputs=**  RndMeth=Zero
  Sum1 : Sum  Inputs=|++
  unitNeg : Gain  Gain=-1  ParamDataTypeStr=single
  psiMul3p : Outport  VectorParamsAs1DForOutWhenUnconnected=off
  LqsubLdId : Outport  Port=2
  psi : Outport  Port=3
  wires:
  Product2/1 -> psiMul3p/1
  unitNeg/1 -> Product1/2
  MCT_LqSubLd/1 -> Product1/1
  MCT_IsdDes/1 -> unitNeg/1
  MCT_PsiExc/1 -> psi/1, Sum1/2
  Sum1/1 -> Product2/1
  3p/1 -> Product2/2
  Product1/1 -> LqsubLdId/1, Sum1/1

== matlab function FOC/bldc/Subsystem1/AsrPI1 ==
  data: Kp output single; Ki output single; fdb input; KpHi input; KiHi input; KpLo input; KiLo input; rpm_Lo input; rpm_Hi input
function [Kp,Ki]   = fcn(fdb,KpHi,KiHi,KpLo,KiLo,rpm_Lo,rpm_Hi)
%
if KiHi == single(0)
    asrKiHi = single(0);
else
    asrKiHi = KiHi;
end

if KiLo == single(0)
    asrKiLo = single(0);
else
    asrKiLo = KiLo;
end

if rpm_Hi >= rpm_Lo
    asr_rpm_Hi = rpm_Hi;
    asr_rpm_Lo = rpm_Lo;
else
    asr_rpm_Hi = rpm_Lo;
    asr_rpm_Lo = rpm_Hi;
end

if fdb >= asr_rpm_Hi
    Kp = KpHi;
    Ki = asrKiHi;
elseif fdb <= asr_rpm_Lo
    Kp = KpLo;
    Ki = asrKiLo;
else
    Kp = (KpHi - KpLo)*(fdb - asr_rpm_Lo)/(asr_rpm_Hi - asr_rpm_Lo) + KpLo;
    Ki = (asrKiHi - asrKiLo)*(fdb - asr_rpm_Lo)/(asr_rpm_Hi - asr_rpm_Lo) + asrKiLo;
end

== stateflow chart FOC/bldc/PMC_IsDesCalc/FWC/Chart1 ==
  state PID
    en:
    integ=0;
    du:
    out=kp*err+integ;
    if out>max
    out=max;
    if(err<0)
    integ=integ+ki*err;
    end
    elseif out<min
    out=min;
    if(err>0)
    integ=integ+ki*err;
    end
    else
    integ=integ+ki*err;
    end
    if integ>max
    integ=max;
    elseif integ <min
    integ=min;
    end
  (default) -> PID
  data: err input single; kp input single; ki input single; out output single; integ local single; max input single; min input single; f32_max input single =0.15

== matlab function FOC/bldc/PMC_IsDesCalc/FWC/MATLAB Function1 ==
  data: err input single; out output single; kp input single; ki input single; MAX input single; MIN input single; intg input single; intg output
function [out,intg] = fcn(err,kp,ki,MAX,MIN,intg)
temp = err*kp;
out = temp + intg;
if(out>MAX)
    out = MAX;
    if(err<0)
        intg = intg + ki*err;
    end
elseif(out < MIN)
        out = MIN;
        if(err>0)
            intg = intg + ki*err;
        end
else
    intg = intg + ki*err;
end
max(intg,MIN);
min(intg,MAX);

== matlab function FOC/bldc/MATLAB Function1 ==
  data: speedref input; y output; LpfCoef input; spdswitch input
function y = fcn(speedref,LpfCoef,spdswitch)

if(speedref<=abs(single(spdswitch)))

    y=LpfCoef;
else
    y=single(1);
end

== matlab function FOC/bldc/MATLAB Function ==
  data: uqlimit output; UqPoslimt output; UqNeglimt output; uqlimit_1 input; usd_output output; usq_output output; Drive input; iqref input; iqact input; idref input; idact input; omega input; Ld input; Lq input; psi input; Vdc input; decouple_gain input; ffw_gain input; acr_kp input; acr_ki input; sample_time input; kc input; d_axis_pid_out input; f32_P_Modulation input; d_integral input; q_integral input single; d_integral output; q_integral output; q_decouple_Add_ffw output; d_decouple output; ToSee_idAnti_windup output; ToSee_iqAnti_windup output
function [uqlimit,UqPoslimt,UqNeglimt,usd_output,usq_output,d_integral, q_integral,q_decouple_Add_ffw,d_decouple,ToSee_idAnti_windup,ToSee_iqAnti_windup]  = fcn(uqlimit_1,Drive,iqref,iqact,idref,idact,omega,Ld,Lq,psi,Vdc,decouple_gain,ffw_gain,acr_kp,acr_ki,sample_time,kc,d_axis_pid_out,f32_P_Modulation,d_integral,q_integral)



%persistent temp_d_integral;
persistent reset;
if isempty(reset)
    reset = boolean(1);
    %modulation_state = single(0);
    q_integral = single(0);
    d_integral = single(0);
    %modulation_state_new = single(0);
end


if(Drive==1)
act_Kp= single((sqrt(3)* acr_kp)/Vdc);
act_Ki= single((sqrt(3)* acr_ki*sample_time)/Vdc);
anti_sat_term = (act_Kp * kc * omega) *sample_time;

id_error = single(idref - idact);
iq_error = single(iqref - iqact);


%%%%%%%%%%%%%%%%%%%%%%%%%%d_axle%%%%%%%%%%%%%%%%%%%%%%%%%%%%%%%
d_decouple = (-(omega *Lq*iqref*decouple_gain)*sqrt(3))/Vdc;



UdPoslimt = f32_P_Modulation -d_decouple;  %上限
UdNeglimt = -f32_P_Modulation -d_decouple;  %下限

integral_delta = act_Ki * id_error;   %求当前拍积分
d_integral = d_integral + integral_delta;  %累加
pi_d_AxleOutput=act_Kp*id_error +d_integral;  %求d轴PI总输出

if(pi_d_AxleOutput >UdPoslimt)  %总输出超过上限
    pi_d_AxleOutput = UdPoslimt;  %限幅
  if(id_error<0)  %上限饱和
      temp_idAnti_windup = (-(anti_sat_term * iq_error)) + (id_error * act_Ki);%饱和计算
      if(temp_idAnti_windup >0)  %针对上限饱和的 Anti_windup项必须为正，否则发散
        temp_idAnti_windup = single(0);    
      end
     d_integral= d_integral +temp_idAnti_windup ;
  end
   temp_idAnti_windup = single(0);
   
elseif(pi_d_AxleOutput < UdNeglimt)
  pi_d_AxleOutput = UdNeglimt;

  if(id_error >0 )
        temp_idAnti_windup = (-(anti_sat_term * iq_error)) + (id_error * act_Ki);
      if(temp_idAnti_windup <0)
        temp_idAnti_windup = single(0);    
      end
     d_integral= d_integral +temp_idAnti_windup ;
  end
   temp_idAnti_windup = single(0);
   
else
  temp_idAnti_windup = single(0);
end

ToSee_idAnti_windup = temp_idAnti_windup;


usd_output = pi_d_AxleOutput+d_decouple;
%%%%%%%%%%%%%%%%%%%%%%%%%%限幅值%%%%%%%%%%%%%%%%%%%%%%%%%%%%%%%

temp1 =  single(1.177225) - usd_output*usd_output;
temp1 = sqrt(temp1);
if(temp1 <0)
   temp1 =single(0);
end
temp2 = single(0.1)*single(temp1)+single(0.9)*uqlimit_1;

if(temp2 >f32_P_Modulation)
temp2 = f32_P_Modulation;
end
uqlimit = temp2 ;

%%%%%%%%%%%%%%%%%%%%%%%%%%q_axle%%%%%%%%%%%%%%%%%%%%%%%%%%%%%%%
q_decouple = ((omega *Ld*idref*decouple_gain)*sqrt(3));
q_ffw= omega *psi *ffw_gain*sqrt(2);

q_decouple_Add_ffw= (q_decouple+q_ffw)/Vdc;

UqPoslimt = uqlimit - q_decouple_Add_ffw;
UqNeglimt = -uqlimit - q_decouple_Add_ffw ;


%integral_delta_q = act_Ki * iq_error;
%q_integral = q_integral + integral_delta_q;

pi_q_AxleOutput=act_Kp*iq_error +q_integral;  %求q轴PI总输出

%%%%%%%%%%%%%%%%%%%%%%%%%%q_axle积分器限幅值%%%%%%%%%%%%%%%%%%%%%%%%%%%%%%%

if(pi_q_AxleOutput >UqPoslimt)  %总输出超过上限
    integral_delta_q = single(0);  %限幅
  if(iq_error<0)  %上限饱和
      temp_iqAnti_windup = (-(anti_sat_term * id_error)) + (iq_error * act_Ki);%饱和计算
      if(temp_iqAnti_windup >0)  %针对上限饱和的 Anti_windup项必须为正，否则发散
        temp_iqAnti_windup = single(0);
      end
  else
      temp_iqAnti_windup= single(0);
  end
 
elseif(pi_q_AxleOutput < UqNeglimt)
  integral_delta_q = single(0);

  if(iq_error >0 )
        temp_iqAnti_windup = (-(anti_sat_term * id_error)) + (iq_error * act_Ki);
      if(temp_iqAnti_windup <0)
        temp_iqAnti_windup = single(0);    
      end
  else
      temp_iqAnti_windup= single(0);
  end
   

else
  temp_iqAnti_windup = single(0);
  integral_delta_q = act_Ki * iq_error;
  
end
q_integral = q_integral +integral_delta_q+temp_iqAnti_windup;  
ToSee_iqAnti_windup = temp_iqAnti_windup;

 if(q_integral >UqPoslimt)  %总输出超过上限
 q_integral = UqPoslimt;
 elseif(q_integral <UqNeglimt)
 q_integral = UqNeglimt;
 else

 end

 if(act_Kp*iq_error+q_integral>UqPoslimt)
     Q_Axle_final = UqPoslimt;
 elseif(act_Kp*iq_error+q_integral<UqNeglimt)
     Q_Axle_final = UqNeglimt;
 else
     Q_Axle_final =act_Kp*iq_error+q_integral;
 end

usq_output = Q_Axle_final +q_decouple_Add_ffw;
%%%%%%%%%%%%%%%%%%%%%%%%%%%%%%%%%%%%%%%%%%%%%%%%%%%%%%%%%
else
    q_integral = single(0);
    d_integral = single(0);
    usd_output = single(0);
    usq_output = single(0);
    q_decouple_Add_ffw = single(0);
    d_decouple = single(0);
    uqlimit = single(0);
    UqPoslimt = single(0);
    UqNeglimt = single(0);
    ToSee_idAnti_windup =single(0);
    ToSee_iqAnti_windup =single(0);
end
